simulink model "two_blocks_w_spring_v0"  (R2016b)
settings: Solver=VariableStepAuto  StartTime=0.0  StopTime=100.0  RelTol=1e-3
settings Model: Creator=ixohoxi  LastModifiedBy=ixohoxi

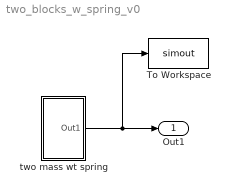
== system two_blocks_w_spring_v0 ==
  To Workspace : ToWorkspace  VariableName=simout  SaveFormat=Timeseries  SampleTime=-1
  two mass wt spring : Subsystem  mask{m_h=1, m_v=0.5, d_e=0.5, g=9.8, mu_h=0.1, mu_v=0.2, k=5}
      mask prompts: m_h "horizontal mass"; m_v "vertical mass"; d_e "spring equilibrium position"; g "gavitational"; mu_h "horizontal friction"; mu_v "vertical friction"; k "spring constant"
  Out1 : Outport
  wires:
  two mass wt spring/1(Out1) -> To Workspace/1, Out1/1

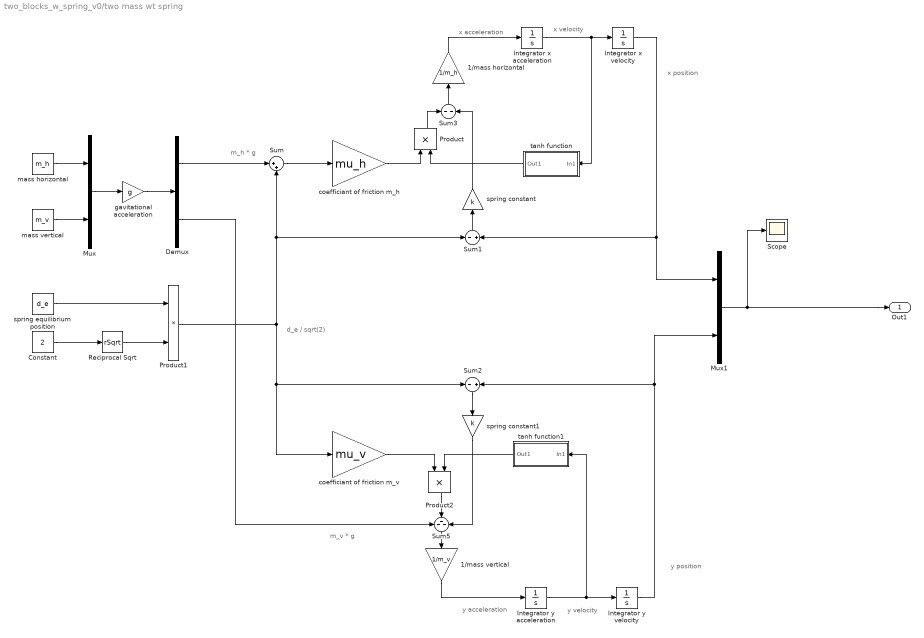
== system two_blocks_w_spring_v0/two mass wt spring ==
  note: m_v * g
  note: m_h * g
  note: d_e / sqrt(2)
  note: x position
  note: x acceleration
  note: x velocity
  note: y position
  note: y acceleration
  note: y velocity
  " spring constant" : Gain  Gain=k
  " spring constant1" : Gain  Gain=k
  1/mass horizontal : Gain  Gain=1/m_h
  1/mass vertical : Gain  Gain=1/m_v
  Constant : Constant  Value=2
  Demux : Demux  Outputs=2
  Integrator x acceleration : Integrator
  Integrator x velocity : Integrator
  Integrator y acceleration : Integrator
  Integrator y velocity : Integrator
  Mux : Mux  Inputs=2
  Mux1 : Mux  Inputs=2
  Product : Product
  Product1 : Product
  Product2 : Product
  Reciprocal Sqrt : Sqrt  Operator=rSqrt  SaturateOnIntegerOverflow=on
  Scope : Scope
  Sum : Sum  Inputs=|++
  Sum1 : Sum  Inputs=-+
  Sum2 : Sum  Inputs=-+
  Sum3 : Sum  Inputs=--
  Sum5 : Sum  Inputs=---
  "coefficiant of friction m_h " : Gain  Gain=mu_h
  coefficiant of friction m_v : Gain  Gain=mu_v
  gavitational acceleration : Gain  Gain=g
  "mass horizontal " : Constant  Value=m_h
  mass vertical : Constant  Value=m_v
  spring equilibrium position : Constant  Value=d_e
  tanh function : Subsystem  mask{a=20}
      mask prompts: a "growth factor"
  tanh function1 : Subsystem  mask{a=20}
      mask prompts: a "growth factor"
  Out1 : Outport
  wires:
  Product/1 -> Sum3/1
  "coefficiant of friction m_h "/1 -> Product/1
  1/mass vertical/1 -> Integrator y acceleration/1
  Mux/1 -> gavitational acceleration/1
  Sum/1 -> "coefficiant of friction m_h "/1
  Product2/1 -> Sum5/2
  Integrator y velocity/1 -> Mux1/2, Sum2/2
  Integrator x acceleration/1 -> tanh function/1(In1), Integrator x velocity/1
  gavitational acceleration/1 -> Demux/1
  tanh function/1(Out1) -> Product/2
  mass vertical/1 -> Mux/2
  Demux/1 -> Sum/1
  "mass horizontal "/1 -> Mux/1
  Integrator y acceleration/1 -> Integrator y velocity/1, tanh function1/1(In1)
  Product1/1 -> Sum2/1, coefficiant of friction m_v/1, Sum1/1, Sum/2
  spring equilibrium position/1 -> Product1/1
  Reciprocal Sqrt/1 -> Product1/2
  Constant/1 -> Reciprocal Sqrt/1
  1/mass horizontal/1 -> Integrator x acceleration/1
  Integrator x velocity/1 -> Sum1/2, Mux1/1
  Sum3/1 -> 1/mass horizontal/1
  Demux/2 -> Sum5/1
  coefficiant of friction m_v/1 -> Product2/1
  tanh function1/1(Out1) -> Product2/2
  Mux1/1 -> Scope/1, Out1/1
  Sum5/1 -> 1/mass vertical/1
  Sum1/1 -> " spring constant"/1
  " spring constant"/1 -> Sum3/2
  Sum2/1 -> " spring constant1"/1
  " spring constant1"/1 -> Sum5/3

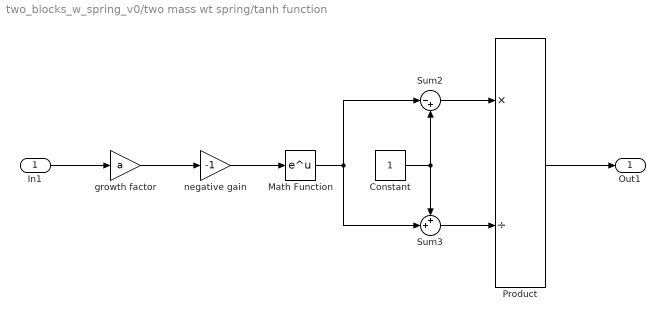
== system two_blocks_w_spring_v0/two mass wt spring/tanh function ==
  In1 : Inport
  Constant : Constant
  Math Function : Math  SaturateOnIntegerOverflow=on
  Product : Product  Inputs=*/
  Sum2 : Sum  Inputs=|-+
  Sum3 : Sum  Inputs=++|
  growth factor : Gain  Gain=a
  negative gain : Gain  Gain=-1
  Out1 : Outport
  wires:
  Sum2/1 -> Product/1
  Math Function/1 -> Sum3/2, Sum2/1
  Product/1 -> Out1/1
  Sum3/1 -> Product/2
  Constant/1 -> Sum3/1, Sum2/2
  In1/1 -> growth factor/1
  growth factor/1 -> negative gain/1
  negative gain/1 -> Math Function/1

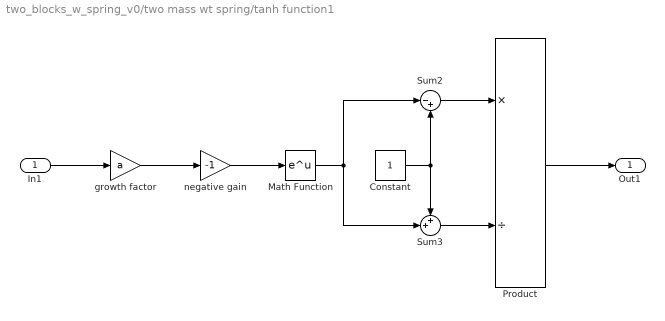
== system two_blocks_w_spring_v0/two mass wt spring/tanh function1 ==
  In1 : Inport
  Constant : Constant
  Math Function : Math  SaturateOnIntegerOverflow=on
  Product : Product  Inputs=*/
  Sum2 : Sum  Inputs=|-+
  Sum3 : Sum  Inputs=++|
  growth factor : Gain  Gain=a
  negative gain : Gain  Gain=-1
  Out1 : Outport
  wires:
  Sum2/1 -> Product/1
  Math Function/1 -> Sum3/2, Sum2/1
  Product/1 -> Out1/1
  Sum3/1 -> Product/2
  Constant/1 -> Sum3/1, Sum2/2
  In1/1 -> growth factor/1
  growth factor/1 -> negative gain/1
  negative gain/1 -> Math Function/1
